simulink model "DEPREMSIGNAL_PIV"  (R2024b)
settings: Solver=ode3  StartTime=0.0  StopTime=inf  FixedStep=0.05  RelTol=1e-3  EnableMultiTasking=on
libraries: arduinolib x6, arduinosensorlib x2
settings Model: ExtModeTrigDuration=2  Creator=cagla  LastModifiedBy=Asus
settings SolverCC: AutoInsertRateTranBlk=on
settings DataIOCC: ReturnWorkspaceOutputs=off
settings OptimizationCC: EnhancedBackFolding=on  PassReuseOutputArgsAs=Individual arguments  ZeroExternalMemoryAtStartup=off  ZeroInternalMemoryAtStartup=off  MaxStackSize=64  OptimizeBlockOrder=speed  DifferentSizesBufferReuse=on  OptimizationCustomize=off  EfficientTunableParamExpr=on
settings DebuggingCC: ParameterTunabilityLossMsg=error
settings HardwareCC: ProdBitPerInt=16  ProdBitPerPointer=16  ProdBitPerSizeT=16  ProdBitPerPtrDiffT=16  ProdLargestAtomicFloat=None  ProdWordSize=8  ProdHWDeviceType=Atmel->AVR
settings SFSimCC: MATLABDynamicMemAlloc=off
settings RTWCC: Description=Embedded Coder  SystemTargetFile=ert.tlc  HardwareBoard=Arduino Mega 2560  TemplateMakefile=ert_default_tmf  Toolchain=Arduino AVR  BuildConfiguration=Faster Runs
settings CodeAppCC: ForceParamTrailComments=on  IgnoreCustomStorageClasses=off  OperatorAnnotations=on  SimulinkDataObjDesc=on  SFDataObjDesc=on  InsertBlockDesc=on
settings ERTTargetCC: SupportContinuousTime=on  SupportNonInlinedSFcns=on  SupportVariableSizeSignals=on  ExtModeTransport=3  ExtModeStaticAlloc=on  ExtModeAutomaticAllocSize=off  ExtModeStaticAllocSize=2048  ExtModeMexFile=ext_xcp  ExtModeIntrfLevel=Level2 - Open  InlinedParameterPlacement=Hierarchical

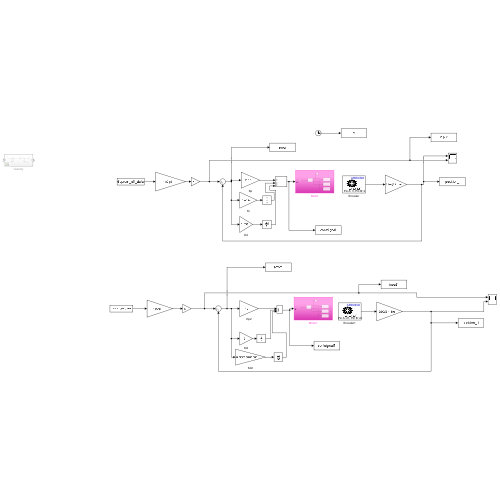
[thumbnail: Simulink's stored preview of the top-level diagram]
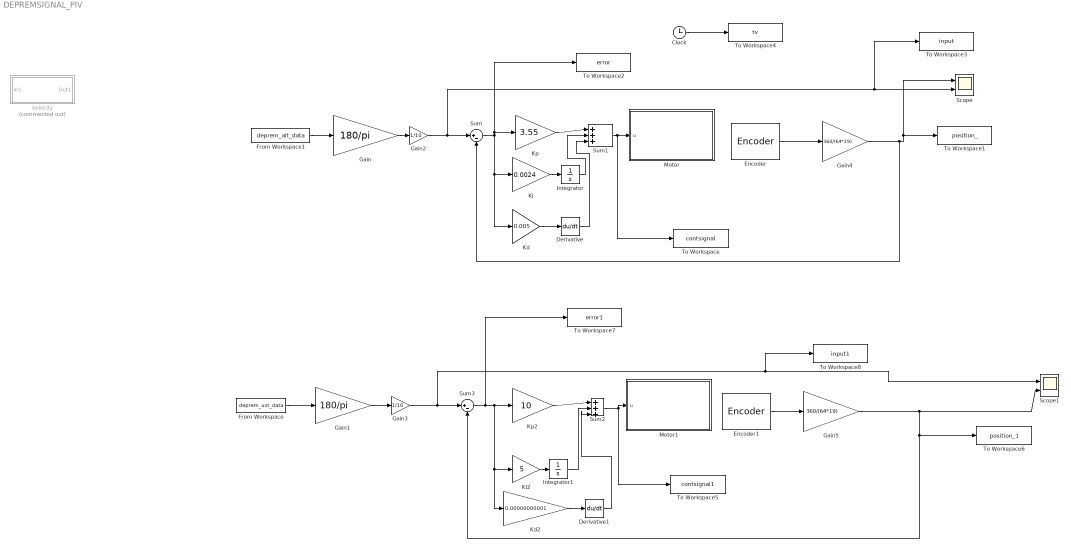
== system DEPREMSIGNAL_PIV ==
  Clock : Clock
  Derivative : Derivative
  Derivative1 : Derivative
  Encoder : arduinosensorlib/Encoder  InputA=3  InputB=2  Mode=No reset  SampleTime=-1
      settings: SourceProductName=Sensors
  Encoder1 : arduinosensorlib/Encoder  InputA=21  InputB=20  Mode=No reset  SampleTime=-1
      settings: SourceProductName=Sensors
  From Workspace : FromWorkspace  VariableName=deprem_ust_data
  From Workspace1 : FromWorkspace  VariableName=deprem_alt_data
  Gain : Gain  Gain=180/pi
  Gain1 : Gain  Gain=180/pi
  Gain2 : Gain  Gain=1/10
  Gain3 : Gain  Gain=1/10
  Gain4 : Gain  Gain=360/(64*19)
  Gain5 : Gain  Gain=360/(64*19)
  Integrator : Integrator
  Integrator1 : Integrator
  Kd : Gain  Gain=0.005
  Kd2 : Gain  Gain=0.00000000001
  Ki : Gain  Gain=0.0024
  Ki2 : Gain  Gain=5
  Kp : Gain  Gain=3.55
  Kp2 : Gain  Gain=10
  Motor : Subsystem
  Motor1 : Subsystem
  Scope : Scope  NumInputPorts=2
  Scope1 : Scope  NumInputPorts=2
  Sum : Sum  Inputs=|+-
  Sum1 : Sum  Inputs=|+++
  Sum2 : Sum  Inputs=|+++
  Sum3 : Sum  Inputs=|+-
  To Workspace : ToWorkspace  VariableName=contsignal  SampleTime=-1
      settings: Save2DSignal=2-D array (concatenate along first dimension)
  To Workspace1 : ToWorkspace  VariableName=position_  SampleTime=-1
      settings: Save2DSignal=2-D array (concatenate along first dimension)
  To Workspace2 : ToWorkspace  VariableName=error  SampleTime=-1
      settings: Save2DSignal=2-D array (concatenate along first dimension)
  To Workspace3 : ToWorkspace  VariableName=input  SampleTime=-1
      settings: Save2DSignal=2-D array (concatenate along first dimension)
  To Workspace4 : ToWorkspace  VariableName=tv  SampleTime=-1
      settings: Save2DSignal=2-D array (concatenate along first dimension)
  To Workspace5 : ToWorkspace  VariableName=contsignal1  SampleTime=-1
      settings: Save2DSignal=2-D array (concatenate along first dimension)
  To Workspace6 : ToWorkspace  VariableName=position_1  SampleTime=-1
      settings: Save2DSignal=2-D array (concatenate along first dimension)
  To Workspace7 : ToWorkspace  VariableName=error1  SampleTime=-1
      settings: Save2DSignal=2-D array (concatenate along first dimension)
  To Workspace8 : ToWorkspace  VariableName=input1  SampleTime=-1
      settings: Save2DSignal=2-D array (concatenate along first dimension)
  Velocity : Subsystem  Commented=on
  wires:
  Sum3/1 -> Kd2/1, Ki2/1, Kp2/1, To Workspace7/1
  Encoder1/1 -> Gain5/1
  Gain4/1 -> Scope/1, To Workspace1/1, Sum/2
  Gain5/1 -> To Workspace6/1, Sum3/2, Scope1/2
  Sum1/1 -> To Workspace/1, Motor/1(u)
  Sum/1 -> To Workspace2/1, Kp/1, Kd/1, Ki/1
  Kp2/1 -> Sum2/1
  Sum2/1 -> Motor1/1(u), To Workspace5/1
  Ki2/1 -> Integrator1/1
  Integrator1/1 -> Sum2/2
  Kd2/1 -> Derivative1/1
  Derivative1/1 -> Sum2/3
  Kp/1 -> Sum1/1
  Integrator/1 -> Sum1/2
  Derivative/1 -> Sum1/3
  Ki/1 -> Integrator/1
  Kd/1 -> Derivative/1
  Encoder/1 -> Gain4/1
  From Workspace1/1 -> Gain/1
  Clock/1 -> To Workspace4/1
  From Workspace/1 -> Gain1/1
  Gain/1 -> Gain2/1
  Gain1/1 -> Gain3/1
  Gain2/1 -> To Workspace3/1, Scope/2, Sum/1
  Gain3/1 -> To Workspace8/1, Scope1/1, Sum3/1

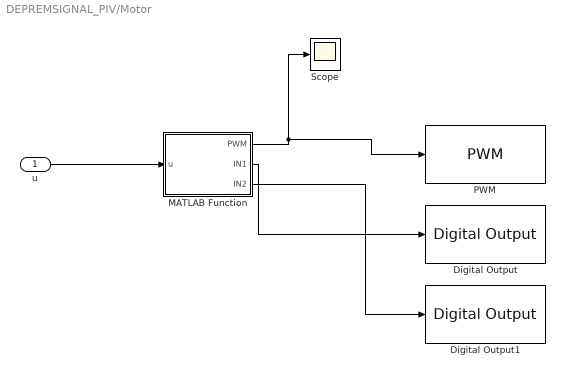
== system DEPREMSIGNAL_PIV/Motor ==
  u : Inport
  Digital Output : arduinolib/Digital Output  pinNumber=8  Direction=output  blockPlatform=arduino
      settings: SourceProductName=Common
  Digital Output1 : arduinolib/Digital Output  pinNumber=7  Direction=output  blockPlatform=arduino
      settings: SourceProductName=Common
  MATLAB Function : MATLAB Function  TreatAsAtomicUnit=on
  PWM : arduinolib/PWM  pinNumber=6  frequencyType=Default  desiredFrequency=490.2  achievableFrequency=490.2
      settings: SourceProductName=Common
  Scope : Scope
  wires:
  MATLAB Function/2(IN1) -> Digital Output/1
  MATLAB Function/1(PWM) -> Scope/1, PWM/1
  MATLAB Function/3(IN2) -> Digital Output1/1
  u/1 -> MATLAB Function/1(u)

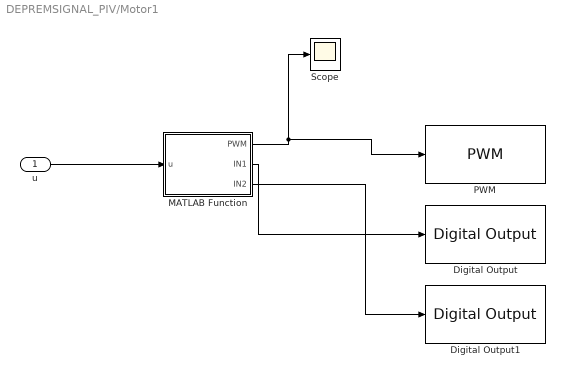
== system DEPREMSIGNAL_PIV/Motor1 ==
  u : Inport
  Digital Output : arduinolib/Digital Output  pinNumber=10  Direction=output  blockPlatform=arduino
      settings: SourceProductName=Common
  Digital Output1 : arduinolib/Digital Output  pinNumber=11  Direction=output  blockPlatform=arduino
      settings: SourceProductName=Common
  MATLAB Function : MATLAB Function  TreatAsAtomicUnit=on
  PWM : arduinolib/PWM  pinNumber=9  frequencyType=Default  desiredFrequency=490.2  achievableFrequency=490.2
      settings: SourceProductName=Common
  Scope : Scope
  wires:
  MATLAB Function/2(IN1) -> Digital Output/1
  MATLAB Function/1(PWM) -> Scope/1, PWM/1
  MATLAB Function/3(IN2) -> Digital Output1/1
  u/1 -> MATLAB Function/1(u)

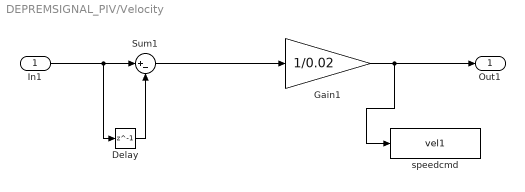
== system DEPREMSIGNAL_PIV/Velocity ==
  In1 : Inport
  Delay : Delay  DelayLength=1
  Gain1 : Gain  Gain=1/0.02
  Sum1 : Sum  Inputs=|+-
  speedcmd : ToWorkspace  VariableName=vel1  SampleTime=-1
      settings: Save2DSignal=2-D array (concatenate along first dimension)
  Out1 : Outport
  wires:
  Gain1/1 -> speedcmd/1, Out1/1
  In1/1 -> Delay/1, Sum1/1
  Sum1/1 -> Gain1/1
  Delay/1 -> Sum1/2

== matlab function DEPREMSIGNAL_PIV/Motor1/MATLAB Function ==
  data: u input; PWM output; IN1 output; IN2 output
function [PWM,IN1,IN2] = fcn(u)
PWM=abs(u);
if u<0
    IN1=1;
    IN2=0;
elseif u>0
    IN1=0;
    IN2=1;
else
    IN1=0;
    IN2=0;
end

== matlab function DEPREMSIGNAL_PIV/Motor/MATLAB Function ==
  data: u input; PWM output; IN1 output; IN2 output
function [PWM,IN1,IN2] = fcn(u)
PWM=abs(u);
if u<0
    IN1=1;
    IN2=0;
elseif u>0
    IN1=0;
    IN2=1;
else
    IN1=0;
    IN2=0;
end
